simulink model "sample_system_OLD"  (R2022a)
settings: Solver=VariableStepAuto  StartTime=0.0  StopTime=20  RelTol=1e-3
values from neighbouring files (symbols this model uses):
  A = load('A.mat').A_bar    [Run_sim.m]
  attack_start_injection = 2    [Run_sim.m]
  B = load('B.mat').B_bar    [Run_sim.m]
  C = load('C.mat').C_obsv    [Run_sim.m]    (also in generator_example_concentric_circles_discriminators.m = colororder)
  Cc = ones(1,n_states)    [Run_sim.m]
  detection_start = 1    [Run_sim.m]
  K = place(A,B,Pc)    [Run_sim.m]
  L = place(A.',C.',Po).'    [Run_sim.m]    (also in detection.m = size(r,1); effectiveness.m = size(critical_meas,1))
  x0 = rand(n_states,1)    [Run_sim.m]
  x_hat0 = x0    [Run_sim.m]
libraries: simulink x1
settings Model: Creator=Abelb  LastModifiedBy=Anubi
settings DebuggingCC: UnconnectedInputMsg=warning  UnconnectedOutputMsg=warning  UnconnectedLineMsg=warning
settings RTWCC: DLArmComputeVersion=19.05

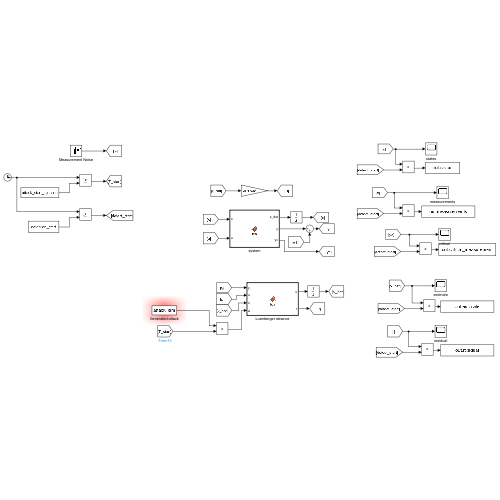
[thumbnail: Simulink's stored preview of the top-level diagram]
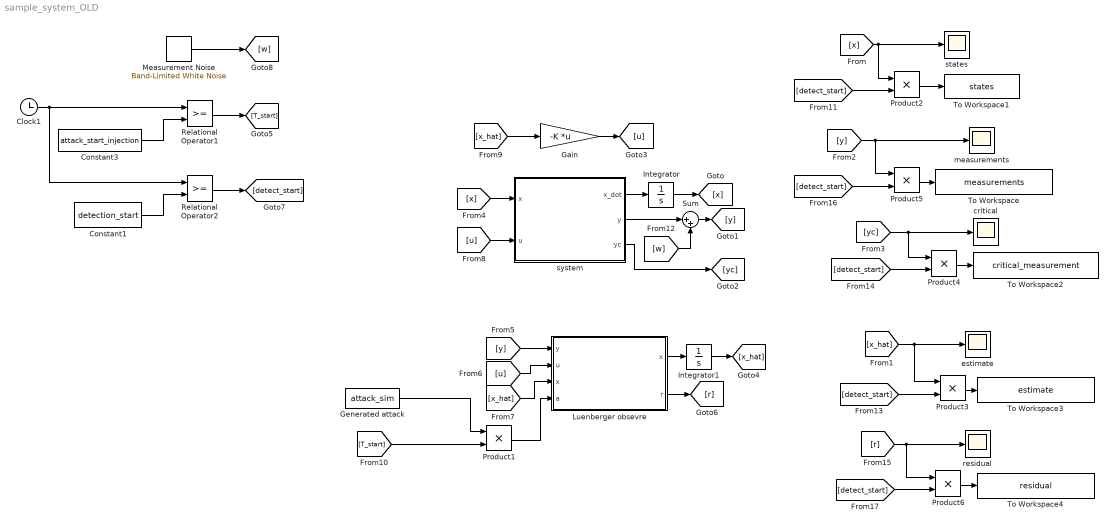
== system sample_system_OLD ==
  Clock1 : Clock
  Constant1 : Constant  Value=detection_start
  Constant3 : Constant  Value=attack_start_injection
  Gain : Gain  Gain=-K  Multiplication=Matrix(K*u) (u vector)
  Generated attack : FromWorkspace  VariableName=attack_sim  OutputAfterFinalValue=Holding final value
  Integrator : Integrator  InitialCondition=x0
  Integrator1 : Integrator  InitialCondition=x_hat0
  Luenberger obsevre : MATLAB Function  TreatAsAtomicUnit=on
  Measurement Noise : simulink/Sources/Band-Limited White Noise  Cov=[0.0001]  Ts=0.1  seed=[23341]
  Product{1..6} (6 alike) : Product
  Relational Operator1 : RelationalOperator  OutDataTypeStr=boolean  RndMeth=Simplest  InputSameDT=off
  Relational Operator2 : RelationalOperator  OutDataTypeStr=boolean  RndMeth=Simplest  InputSameDT=off
  Sum : Sum  Inputs=|++
  To Workspace : ToWorkspace  VariableName=measurements  SaveFormat=Timeseries  SampleTime=-1
  To Workspace1 : ToWorkspace  VariableName=states  SaveFormat=Timeseries  SampleTime=-1
  To Workspace2 : ToWorkspace  VariableName=critical_measurement  SaveFormat=Timeseries  SampleTime=-1
  To Workspace3 : ToWorkspace  VariableName=estimate  SaveFormat=Timeseries  SampleTime=-1
  To Workspace4 : ToWorkspace  VariableName=residual  SaveFormat=Timeseries  SampleTime=-1
  critical : Scope
  estimate : Scope
  measurements : Scope
  residual : Scope
  states : Scope
  system : MATLAB Function  TreatAsAtomicUnit=on
  wires:
  system/1(x_dot) -> Integrator/1
  Integrator/1 -> [x]
  [x_hat] -> Gain/1
  [x] -> Product2/1, states/1
  system/3(yc) -> [yc]
  [x] -> system/1(x)
  [y] -> Luenberger obsevre/1(y)
  Gain/1 -> [u]
  [u] -> Luenberger obsevre/2(u)
  Luenberger obsevre/1(x) -> Integrator1/1
  Integrator1/1 -> [x_hat]
  [x_hat] -> Luenberger obsevre/3("x ")
  [u] -> system/2(u)
  Clock1/1 -> Relational Operator1/1, Relational Operator2/1
  Constant3/1 -> Relational Operator1/2
  Relational Operator1/1 -> [T_start]
  [T_start] -> Product1/2
  Product2/1 -> To Workspace1/1
  [y] -> Product5/1, measurements/1
  [yc] -> Product4/1, critical/1
  [x_hat] -> Product3/1, estimate/1
  Luenberger obsevre/2(r) -> [r]
  [r] -> Product6/1, residual/1
  [detect_start] -> Product6/2
  Relational Operator2/1 -> [detect_start]
  Constant1/1 -> Relational Operator2/2
  Measurement Noise/1 -> [w]
  Sum/1 -> [y]
  [w] -> Sum/2
  system/2(y) -> Sum/1
  Product1/1 -> Luenberger obsevre/4(a)
  Generated attack/1 -> Product1/1
  Product6/1 -> To Workspace4/1
  [detect_start] -> Product3/2
  Product3/1 -> To Workspace3/1
  [detect_start] -> Product4/2
  Product4/1 -> To Workspace2/1
  [detect_start] -> Product5/2
  Product5/1 -> To Workspace/1
  [detect_start] -> Product2/2

== matlab function sample_system_OLD/Luenberger obsevre ==
  data: y input; u input; x output; x input; a input; A parameter; C parameter; B parameter; L parameter; r output
function [x,r] = fcn(y,u,x,a,A, C, B,L)

x = A*x+B*u + L*(y+a-C*x);
r = norm(y+a-C*x);

== matlab function sample_system_OLD/system ==
  data: x_dot output; x input; u input; y output; yc output; A parameter; Cc parameter; C parameter; B parameter
function [x_dot,y,yc] = fcn(x,u,A,Cc, C, B)

x_dot = A*x + B*u;
y = C*x;
yc = Cc*x;
